simulink model "Subsystem"  (R2020a)
settings: Solver=VariableStepAuto  StartTime=0.0  StopTime=10.0  RelTol=1e-3
model workspace (MAT data in the model file):
  K = Simulink.Parameter
  K.Value = 3
  K.DataType = 'auto'
  K.Dimensions = [1 1]
  L = Simulink.Parameter
  L.Value = -4
  L.DataType = 'auto'
  L.Dimensions = [1 1]
  M = Simulink.Parameter
  M.Value = -5
  M.DataType = 'auto'
  M.Dimensions = [1 1]
  N = Simulink.Parameter
  N.Value = 6
  N.DataType = 'auto'
  N.Dimensions = [1 1]
settings Model: Creator=Riyansh  LastModifiedBy=Riyansh
settings DataIOCC: SaveOutput=off  SaveTime=off

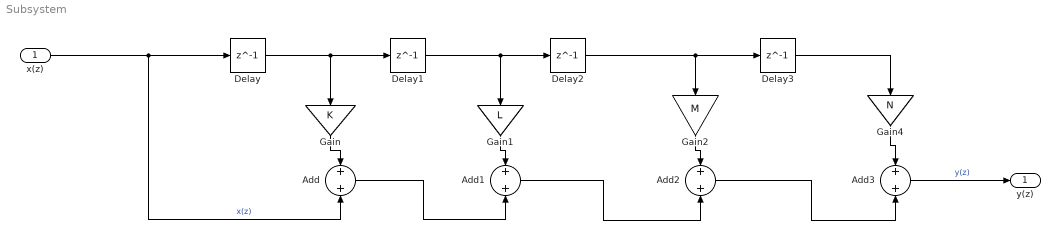
== system Subsystem ==
  x(z) : Inport  OutDataTypeStr=double  PortDimensions=1  SampleTime=[0,1]
  Add{,1..3} (4 alike) : Sum
  Delay{,1..3} (4 alike) : Delay  DelayLength=1  InitialCondition=0
  Gain : Gain  Gain=K
  Gain1 : Gain  Gain=L
  Gain2 : Gain  Gain=M
  Gain4 : Gain  Gain=N
  y(z) : Outport  OutDataTypeStr=double  PortDimensions=1  SampleTime=[0,1]
  wires:
  Delay3/1 -> Gain4/1
  Gain1/1 -> Add1/1
  Add2/1 -> Add3/2
  Delay1/1 -> Gain1/1, Delay2/1
  Add1/1 -> Add2/2
  x(z)/1 -> Delay/1, Add/2  "x(z)"
  Gain2/1 -> Add2/1
  Add/1 -> Add1/2
  Gain/1 -> Add/1
  Delay/1 -> Gain/1, Delay1/1
  Gain4/1 -> Add3/1
  Delay2/1 -> Gain2/1, Delay3/1
  Add3/1 -> y(z)/1  "y(z)"
